simulink model "pedal_with_SIL_test"  (R2021a)
settings: Solver=FixedStepDiscrete  StartTime=0.0  StopTime=10.0  FixedStep=1e-3  RelTol=1e-3
undefined symbols (not defined in the file or in its folder): sigbuilder_block
libraries: pil_lib x1
settings Model: Creator=Beshary  LastModifiedBy=Beshary
settings DataIOCC: OutputSaveName=MIL_out  LoggingToFile=on
settings OptimizationCC: DefaultParameterBehavior=Inlined  UseDivisionForNetSlopeComputation=on  GainParamInheritBuiltInType=on  UseFloatMulNetSlope=on  InlineInvariantSignals=on  PassReuseOutputArgsAs=Individual arguments  ZeroExternalMemoryAtStartup=off  ZeroInternalMemoryAtStartup=off  NoFixptDivByZeroProtection=on  EfficientFloat2IntCast=on  LifeSpan=1  OptimizeBlockOrder=speed  DifferentSizesBufferReuse=on  EfficientTunableParamExpr=on
settings DebuggingCC: ParameterTunabilityLossMsg=error
settings HardwareCC: ProdBitPerPointer=32  ProdBitPerSizeT=32  ProdBitPerPtrDiffT=32  ProdLargestAtomicInteger=Long  ProdLargestAtomicFloat=Double  ProdWordSize=32  ProdLongLongMode=on  ProdHWDeviceType=ARM Compatible->ARM Cortex-M
settings SFSimCC: MATLABDynamicMemAlloc=off
settings RTWCC: SystemTargetFile=ert.tlc  TemplateMakefile=ert_default_tmf
settings CodeAppCC: ForceParamTrailComments=on  IgnoreCustomStorageClasses=off  OperatorAnnotations=on  SimulinkDataObjDesc=on  SFDataObjDesc=on  CustomSymbolStrGlobalVar=rt$N$M  CustomSymbolStrType=$N$M  CustomSymbolStrFcn=$N$M$F  CustomSymbolStrMacro=$N$M  InsertBlockDesc=on
settings ERTTargetCC: TargetLangStandard=C99 (ISO)  GenerateSampleERTMain=on  IncludeMdlTerminateFcn=off  CombineSignalStateStructs=on  SuppressErrorStatus=on  SupportAbsoluteTime=off  SupportComplex=off  InlinedParameterPlacement=NonHierarchical  ERTCustomFileTemplate=example_file_process.tlc  ERTFilePackagingFormat=CompactWithDataFile

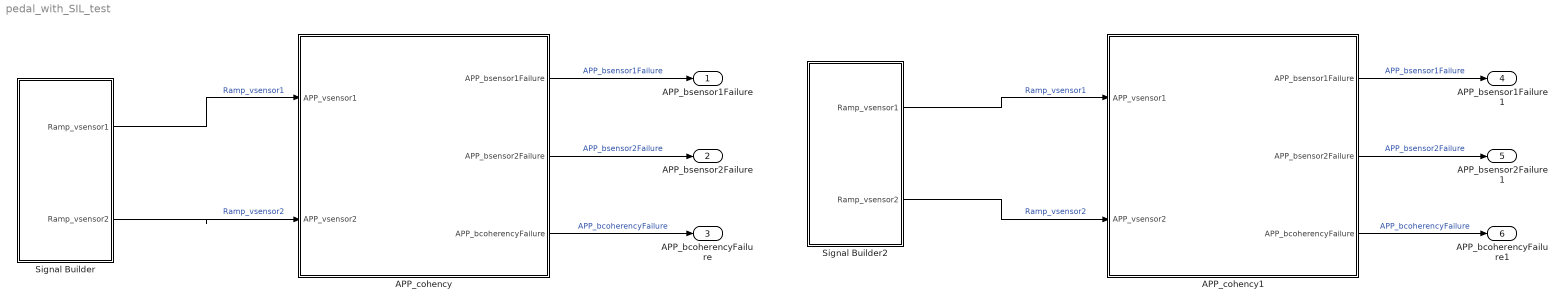
== system pedal_with_SIL_test ==
  APP_cohency : Subsystem  TreatAsAtomicUnit=on
  APP_cohency1 : Subsystem  Tag=__SL_testing_harness_stub_  DialogController=pil_create_dialog  LoadFcn=|
      | try
      |    if ~strcmp(rtw.pil.getPILVersion, '9.10 (R2021a)_15')
      |       set_param(gcb, 'DialogController', '');
      |       set_param(gcb, 'DialogControllerArgs', '');
      |    end
      | catch e
      |       set_param(gcb, 'DialogController', '');
      |       set_param(gcb, 'DialogControllerArgs', '');
      | end
      mask help: PIL:pil:XILBlockMaskDesc
      mask Display: disp('SIL');
  Signal Builder : Subsystem  Tag=STV Subsys  LoadFcn=sigbuilder_block('load');  StartFcn=sigbuilder_block('start');  StopFcn=sigbuilder_block('stop');  ClipboardFcn=sigbuilder_block('clipboard');  mask(Sigbuilder block){tuvar=[0:10]}
      mask help: Simulink:masks:SigbuilderBlock_MD
      mask init:
      | if ~strcmp(get_param(bdroot(gcbh),'SimulationStatus'),'stopped') tuvar = sigbuilder_block('maskInit'); end
      settings: CopyFcn=sigbuilder_block('copy');  DeleteFcn=sigbuilder_block('delete');  ModelCloseFcn=sigbuilder_block('modelClose');  PreSaveFcn=sigbuilder_block('preSave');  PauseFcn=sigbuilder_block('pause');  ContinueFcn=sigbuilder_block('continue');  NameChangeFcn=sigbuilder_block('namechange');  OpenFcn=sigbuilder_block('open',[437.6 146.4 550.4 400.2 ]);  CloseFcn=sigbuilder_block('close');
      mask Display: plot(0, 0, 100, 100,[2, 2, 32, 32, 2], [68, 8, 8, 68, 68],[32, 2], [38, 38], [32, 19, 2],[53, 60, 44], [32, 17, 17, 2],[16, 16, 31, 31]);txt = getActiveGroup(gcbh);text(2, 100, txt,'verticalAlignment', 'top');
  Signal Builder2 : Subsystem  Tag=STV Subsys  LoadFcn=sigbuilder_block('load');  StartFcn=sigbuilder_block('start');  StopFcn=sigbuilder_block('stop');  ClipboardFcn=sigbuilder_block('clipboard');  mask(Sigbuilder block){tuvar=[0:10]}
      mask help: Simulink:masks:SigbuilderBlock_MD
      mask init:
      | if ~strcmp(get_param(bdroot(gcbh),'SimulationStatus'),'stopped') tuvar = sigbuilder_block('maskInit'); end
      settings: CopyFcn=sigbuilder_block('copy');  DeleteFcn=sigbuilder_block('delete');  ModelCloseFcn=sigbuilder_block('modelClose');  PreSaveFcn=sigbuilder_block('preSave');  PauseFcn=sigbuilder_block('pause');  ContinueFcn=sigbuilder_block('continue');  NameChangeFcn=sigbuilder_block('namechange');  OpenFcn=sigbuilder_block('open',[437.6 146.4 550.4 400.2 ]);  CloseFcn=sigbuilder_block('close');
      mask Display: plot(0, 0, 100, 100,[2, 2, 32, 32, 2], [68, 8, 8, 68, 68],[32, 2], [38, 38], [32, 19, 2],[53, 60, 44], [32, 17, 17, 2],[16, 16, 31, 31]);txt = getActiveGroup(gcbh);text(2, 100, txt,'verticalAlignment', 'top');
  APP_bsensor1Failure : Outport
  APP_bsensor2Failure : Outport  Port=2
  APP_bcoherencyFailure : Outport  Port=3
  APP_bsensor1Failure1 : Outport  Port=4
  APP_bsensor2Failure1 : Outport  Port=5
  APP_bcoherencyFailure1 : Outport  Port=6
  wires:
  Signal Builder/2(Ramp_vsensor2) -> APP_cohency/2(APP_vsensor2)  "Ramp_vsensor2"
  Signal Builder/1(Ramp_vsensor1) -> APP_cohency/1(APP_vsensor1)  "Ramp_vsensor1"
  APP_cohency/3(APP_bcoherencyFailure) -> APP_bcoherencyFailure/1  "APP_bcoherencyFailure"
  APP_cohency/2(APP_bsensor2Failure) -> APP_bsensor2Failure/1  "APP_bsensor2Failure"
  APP_cohency/1(APP_bsensor1Failure) -> APP_bsensor1Failure/1  "APP_bsensor1Failure"
  Signal Builder2/1(Ramp_vsensor1) -> APP_cohency1/1(APP_vsensor1)  "Ramp_vsensor1"
  APP_cohency1/2(APP_bsensor2Failure) -> APP_bsensor2Failure1/1  "APP_bsensor2Failure"
  APP_cohency1/1(APP_bsensor1Failure) -> APP_bsensor1Failure1/1  "APP_bsensor1Failure"
  APP_cohency1/3(APP_bcoherencyFailure) -> APP_bcoherencyFailure1/1  "APP_bcoherencyFailure"
  Signal Builder2/2(Ramp_vsensor2) -> APP_cohency1/2(APP_vsensor2)  "Ramp_vsensor2"

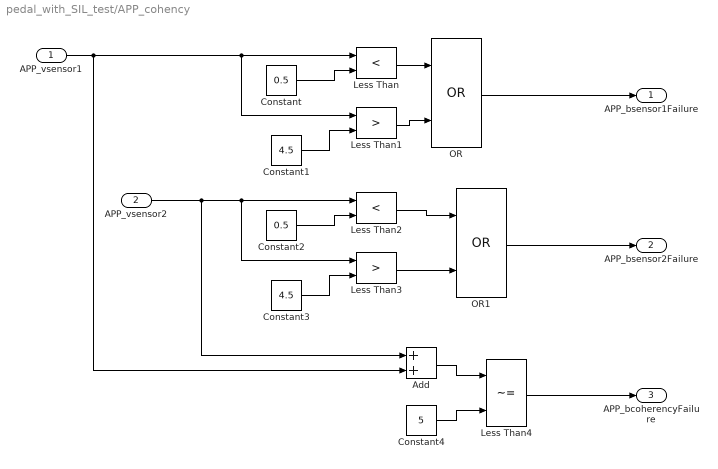
== system pedal_with_SIL_test/APP_cohency ==
  APP_vsensor1 : Inport
  APP_vsensor2 : Inport  Port=2
  Add : Sum
  Constant : Constant  Value=0.5
  Constant1 : Constant  Value=4.5
  Constant2 : Constant  Value=0.5
  Constant3 : Constant  Value=4.5
  Constant4 : Constant  Value=5
  Less Than : RelationalOperator  Operator=<  OutDataTypeStr=boolean  RndMeth=Simplest
  Less Than1 : RelationalOperator  Operator=>  OutDataTypeStr=boolean  RndMeth=Simplest
  Less Than2 : RelationalOperator  Operator=<  OutDataTypeStr=boolean  RndMeth=Simplest
  Less Than3 : RelationalOperator  Operator=>  OutDataTypeStr=boolean  RndMeth=Simplest
  Less Than4 : RelationalOperator  Operator=~=  OutDataTypeStr=boolean  RndMeth=Simplest
  OR : Logic  Operator=OR  AllPortsSameDT=off  OutDataTypeStr=boolean
  OR1 : Logic  Operator=OR  AllPortsSameDT=off  OutDataTypeStr=boolean
  APP_bsensor1Failure : Outport
  APP_bsensor2Failure : Outport  Port=2
  APP_bcoherencyFailure : Outport  Port=3
  wires:
  APP_vsensor1/1 -> Add/2, Less Than1/1, Less Than/1
  Constant/1 -> Less Than/2
  Less Than/1 -> OR/1
  Constant1/1 -> Less Than1/2
  Less Than1/1 -> OR/2
  OR/1 -> APP_bsensor1Failure/1
  Constant3/1 -> Less Than3/2
  Constant2/1 -> Less Than2/2
  APP_vsensor2/1 -> Add/1, Less Than3/1, Less Than2/1
  Less Than2/1 -> OR1/1
  Less Than3/1 -> OR1/2
  OR1/1 -> APP_bsensor2Failure/1
  Add/1 -> Less Than4/1
  Constant4/1 -> Less Than4/2
  Less Than4/1 -> APP_bcoherencyFailure/1

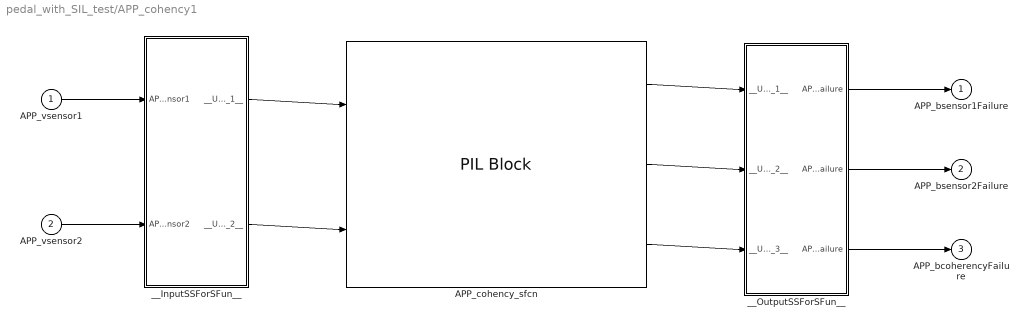
== system pedal_with_SIL_test/APP_cohency1 ==
  APP_vsensor1 : Inport
  APP_vsensor2 : Inport  Port=2
  APP_cohency_sfcn : pil_lib/PIL Block  SimulationMode=SIL  IsTopModelPIL=off  CodeDir=C:\Users\Beshary\Desktop\MBD_OS_DEV\OS_ACDEMY\quiz\Second_Modeling\APP_cohency_ert_rtw  AnchorDir=C:\Users\Beshary\Desktop\MBD_OS_DEV\OS_ACDEMY\quiz\Second_Modeling  ConfigName=Software-in-the-Loop (SIL)  XrelIsTopModelCode=on  XrelIsReusable=off  XrelDWorkNames={}  XrelDWorkTypes={}  XrelModelArgVals={}  XrelOrderedParamNames={}
      settings: SourceProductBaseCode=RT
  __InputSSForSFun__ : Subsystem
  __OutputSSForSFun__ : Subsystem
  APP_bsensor1Failure : Outport
  APP_bsensor2Failure : Outport  Port=2
  APP_bcoherencyFailure : Outport  Port=3
  wires:
  __OutputSSForSFun__/3(APP_bcoherencyFailure) -> APP_bcoherencyFailure/1
  __OutputSSForSFun__/2(APP_bsensor2Failure) -> APP_bsensor2Failure/1
  __OutputSSForSFun__/1(APP_bsensor1Failure) -> APP_bsensor1Failure/1
  APP_cohency_sfcn/3 -> __OutputSSForSFun__/3(__UniqueInportName__3__)
  APP_cohency_sfcn/2 -> __OutputSSForSFun__/2(__UniqueInportName__2__)
  APP_cohency_sfcn/1 -> __OutputSSForSFun__/1(__UniqueInportName__1__)
  __InputSSForSFun__/2(__UniqueOutportName__2__) -> APP_cohency_sfcn/2
  __InputSSForSFun__/1(__UniqueOutportName__1__) -> APP_cohency_sfcn/1
  APP_vsensor2/1 -> __InputSSForSFun__/2(APP_vsensor2)
  APP_vsensor1/1 -> __InputSSForSFun__/1(APP_vsensor1)

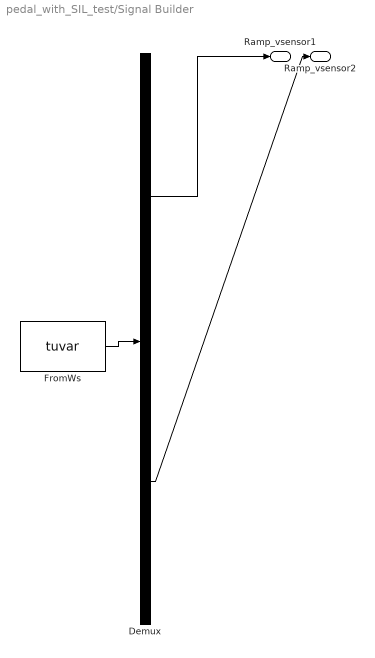
== system pedal_with_SIL_test/Signal Builder ==
  Demux : Demux  Tag=STV Demux  Outputs=2
      settings: DisplayOption=none
  FromWs : FromWorkspace  Tag=STV FromWs  VariableName=tuvar
      SigBuilderData=|
      | common.afterFinalStr = 'Extrapolate'
      | common.sampleTime = 0
      | dataSet.timeRange = [0 13]
      | dataSet.name = 'Sheet1'
      | sbobj.Name = 'Signal Builder'
      | sbobj.Groups.Name = 'Sheet1'
      | sbobj.Groups.Signals(1).Name = 'Ramp_vsensor1'
      | sbobj.Groups.Signals(1).XData = [0 3 3 5 5 7 7 9 9 11 11 13]
      | sbobj.Groups.Signals(1).YData = [4.6 4.6 4.5 4.5 0.5 0.5 0.4 0.4 0.4 0.4 3 3]
      | sbobj.Groups.Signals(2).Name = 'Ramp_vsensor2'
      | sbobj.Groups.Signals(2).XData = [0 3 3 5 5 7 7 9 9 11 11 13]
      | sbobj.Groups.Signals(2).YData = [4.6 4.6 4.5 4.5 4.6 4.6 0.4 0.4 4.6 4.6 0.4 0.4]
      | sbobj.Groups.TimeRange = [0 13]
  Ramp_vsensor1 : Outport  Tag=STV Outport
  Ramp_vsensor2 : Outport  Tag=STV Outport  Port=2
  wires:
  Demux/1 -> Ramp_vsensor1/1
  FromWs/1 -> Demux/1
  Demux/2 -> Ramp_vsensor2/1

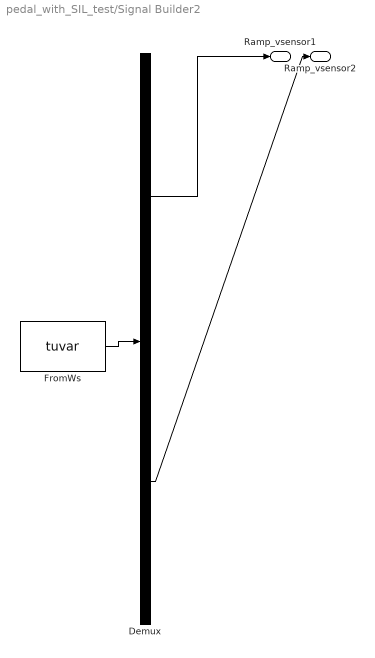
== system pedal_with_SIL_test/Signal Builder2 ==
  Demux : Demux  Tag=STV Demux  Outputs=2
      settings: DisplayOption=none
  FromWs : FromWorkspace  Tag=STV FromWs  VariableName=tuvar
      SigBuilderData=|
      | common.afterFinalStr = 'Extrapolate'
      | common.sampleTime = 0
      | dataSet.timeRange = [0 13]
      | dataSet.name = 'Sheet1'
      | sbobj.Name = 'Signal Builder'
      | sbobj.Groups.Name = 'Sheet1'
      | sbobj.Groups.Signals(1).Name = 'Ramp_vsensor1'
      | sbobj.Groups.Signals(1).XData = [0 3 3 5 5 7 7 9 9 11 11 13]
      | sbobj.Groups.Signals(1).YData = [4.6 4.6 4.5 4.5 0.5 0.5 0.4 0.4 0.4 0.4 3 3]
      | sbobj.Groups.Signals(2).Name = 'Ramp_vsensor2'
      | sbobj.Groups.Signals(2).XData = [0 3 3 5 5 7 7 9 9 11 11 13]
      | sbobj.Groups.Signals(2).YData = [4.6 4.6 4.5 4.5 4.6 4.6 0.4 0.4 4.6 4.6 0.4 0.4]
      | sbobj.Groups.TimeRange = [0 13]
  Ramp_vsensor1 : Outport  Tag=STV Outport
  Ramp_vsensor2 : Outport  Tag=STV Outport  Port=2
  wires:
  Demux/1 -> Ramp_vsensor1/1
  FromWs/1 -> Demux/1
  Demux/2 -> Ramp_vsensor2/1

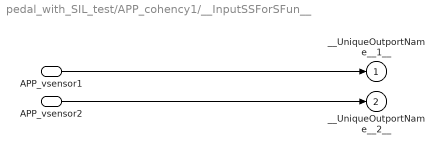
== system pedal_with_SIL_test/APP_cohency1/__InputSSForSFun__ ==
  APP_vsensor1 : Inport
  APP_vsensor2 : Inport  Port=2
  __UniqueOutportName__1__ : Outport
  __UniqueOutportName__2__ : Outport  Port=2
  wires:
  APP_vsensor2/1 -> __UniqueOutportName__2__/1
  APP_vsensor1/1 -> __UniqueOutportName__1__/1

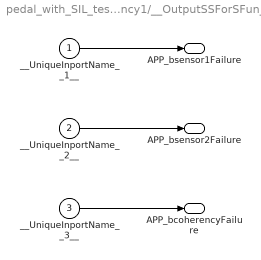
== system pedal_with_SIL_test/APP_cohency1/__OutputSSForSFun__ ==
  __UniqueInportName__1__ : Inport
  __UniqueInportName__2__ : Inport  Port=2
  __UniqueInportName__3__ : Inport  Port=3
  APP_bsensor1Failure : Outport
  APP_bsensor2Failure : Outport  Port=2
  APP_bcoherencyFailure : Outport  Port=3
  wires:
  __UniqueInportName__3__/1 -> APP_bcoherencyFailure/1
  __UniqueInportName__2__/1 -> APP_bsensor2Failure/1
  __UniqueInportName__1__/1 -> APP_bsensor1Failure/1
